simulink model "integration_LQR_model_4"  (R2023a)
settings: Solver=VariableStepAuto  StartTime=0.0  StopTime=30  FixedStep=SampleTime  RelTol=1e-3
PreLoadFcn:
  | %
  | 
  | %   Copyright 2020-2022 The MathWorks, Inc.
  | 
  | %Based on the quadcopter model used in jMAVSim
  | 
  | Ixx = 0.005; %Kgm^2
  | Iyy = 0.005;
  | Izz = 0.009;
  | 
  | 
  | inertia = diag([Ixx, Iyy, Izz]);
  | 
  | mass = 0.8; %Kg
  | g = 9.81; %m/s^2
  | 
  | armLength = 0.33/2; % length of Arm measured from center in m
  | 
  | rotorThrustMax = 4; %N
  | 
  | rotorTorqueMax = 0.05 ;%Nm
  | 
  | rotorTimeConst = 0.005 ;% time constant of rotor (motor + propeller)
  | 
  | %rotorOffset = [0 0 0]; % Rotors position offsets from Gravity center
  | 
  | dragCoeffMov = 0.01; %drag coefficient for linear motion of quadcopter
  | windVel = [0 0 0]';
  | 
  | % Initial states
  | init.posNED = [0, 0, 0]; % m
  | init.vb = [0 0 0]'; %m/s
  | init.euler = [0, 0, 0]'; %Roll Pitch Yaw Rads
  | init.angRates = [0, 0, 0]; %rad/s
  | 
  | 
  | %Computed from above values
  | rotorPositions = zeros(3,4);
  | axisD = armLength/sqrt(2);
  | rotorPositions(:,1) = [axisD, axisD, 0]';
  | rotorPositions(:,2) = [-axisD, -axisD, 0]';
  | rotorPositions(:,3) = [+axisD, -axisD, 0]';
  | rotorPositions(:,4) = [-axisD, axisD, 0]';
  | rotorDir = [-1, -1, 1, 1]; %rotation direction. +ve = clockwise
  | 
  | % Sample Time
  | SampleTime = 0.008;
  | 
  | %Gain to convert m to mm
  | m_to_mm = 1000;
  | 
  | %Gain to convert m/s^2 to mG
  | ms2_to_mg = (1/9.80665)*1000;
  | 
  | %Gain to convert m/s to cm/s
  | ms_to_cms = 100;
  | 
  | %Reference height for 'Flat Earth to LLA'
  | ref_height = -71.3232;
  | 
  | altToPrsGain = 12.0173;
  | altToPrsBias = 101270.95;
  | 
  | % Contact model
  | contact.translation.spring = 3100;
  | contact.translation.damper = 100;
  | contact.translation.friction = 0.5;
  | contact.translation.vd = 0.02;
  | contact.translation.maxFriction = 20;
  | contact.translation.maxNormal = 80;
  | 
  | contact.rotation.spring = 2;
  | contact.rotation.damper = 1;
  | contact.rotation.friction = 0.03;
  | control.rotation.maxMoment = 0.1;
  | control.rotation.friction = 0.025;
  | control.rotation.vd = 0.2;
  | 
  | 
  | %#######################################################
  | % Plant parameters
  | 
  | % Parameters for quadcopter_package_delivery
  | % Copyright 2021-2023 The MathWorks, Inc.
  | 
  | % Size of the ground
  | planex = 12.5;           % m
  | planey = 8.5;            % m
  | planedepth = 0.2;        % m, distance from plane to the reference frame
  | 
  | % Battery Capacity
  | battery_capacity = 7.6*3;
  | 
  | %% Material Property
  | % Assuming the arm of the drone is manufractured by 3D Printing, the ideal
  | % material is PLA, safe, light and cheap, the only concern is its thermal
  | % property
  | rho_pla   = 1.25;            % g/cm^3
  | 
  | % Measured drone mass
  | drone_mass = 1.2726;
  | %% package ground contact properties
  | pkgGrndStiff  = 1000;
  | pkgGrndDamp   = 300;
  | pkgGrndTransW = 1e-3;
  | 
  | 
  | %% Package parameters
  | pkgSize = [1 1 1]*0.14; % m
  | pkgDensity = 1/(pkgSize(1)*pkgSize(2)*pkgSize(3)); % kg/m^3
  | 
  | %% Propeller parameters
  | propeller.diameter = 0.254; % m
  | propeller.Kthrust  = 0.1072;
  | propeller.Kdrag    = 0.01;
  | 
  | air_rho            = 1.225;  % kg/m^3
  | air_temperature    = 273+25; % degK
  | wind_speed         = 0;      % Wind speed (m/s)
  | 
  | %% Leg parameters
  | drone_leg.Extr_Data = flipud([...
  |     0     0;
  |     0.5   0;
  |     1    -1;
  |     0.98 -1;
  |     0.5  -0.02;
  |    -0.5  -0.02;
  |    -0.98 -1;
  |    -1    -1;
  |    -0.5   0].*[1 1]*0.15);
  | 
  | drone_leg.width = 0.01;
  | 
  | %% Motor parameters
  | qc_motor.max_torque = 0.8;  % N*m
  | qc_motor.max_power  = 160;  % W
  | qc_motor.time_const = 0.02; % sec
  | qc_motor.efficiency = 25/30*100; % 0-100
  | qc_motor.efficiency_spd = 5000; % rpm
  | qc_motor.efficiency_trq = 0.05; % N*m
  | qc_motor.rotor_damping  = 1e-7; % N*m/(rad/s)
  | 
  | qc_max_power = qc_motor.max_power;
  | 
  | %% Controller parameters
  | filtM_position = 0.005;
  | kp_position    = 8;
  | ki_position    = 0.04;
  | kd_position    = 3.2;
  | filtD_position = 100;
  | pos2attitude   = 2.4;
  | 
  | filtM_attitude = 0.01;
  | kp_attitude    = 128.505;
  | ki_attitude    = 5.9203;
  | kd_attitude    = 78.2000*2;
  | filtD_attitude = 1000;
  | limit_attitude = 800;
  | 
  | filtM_yaw      = 0.01;
  | kp_yaw         = 25.7010*4*2;
  | ki_yaw         = 5.9203*0.01;
  | kd_yaw         = 78.2000*0.01;
  | filtD_yaw      = 100;
  | limit_yaw      = 20;
  | 
  | filtM_altitude = 0.05;
  | kp_altitude    = 0.27;
  | ki_altitude    = 0.07;
  | kd_altitude    = 0.35;
  | filtD_altitude = 10000;
  | limit_altitude = 10;
  | 
  | kp_motor       = 0.00375;
  | ki_motor       = 4.50000e-4;
  | kd_motor       = 0;
  | filtD_motor    = 10000;
  | filtSpd_motor    = 0.001;
  | limit_motor    = 0.25;
  | 
  | %% Drag coefficients
  | qd_drag.Cd_X = 0.35;
  | qd_drag.Cd_Y = 0.35;
  | qd_drag.Cd_Z = 0.6;
  | qd_drag.Roll = 0.2;
  | qd_drag.Pitch = 0.2;
  | qd_drag.Yaw = 0.2;
  | qd_area.YZ = 0.0875;
  | qd_area.XZ = 0.0900;
  | qd_area.XY = 0.2560;
  | qd_area.Roll = qd_area.XY*2;
  | qd_area.Pitch = qd_area.XY*2;
  | qd_area.Yaw = qd_area.XY;
  | 
  | 
  | waypoints = [-2,-2,0,2,5;-2,-2,0,0,0;0.14,6,6,6,0.14];
values from neighbouring files (symbols this model uses):
  delay_tilt = 0.004    [integration_parameters.m]    (also in simulation_parameters.m)
  kf = 65    [integration_parameters.m]    (also in simulation_parameters.m)
  Lh = 0.2    [CoG_shift.m]    (also in integration_parameters.m; simulation_parameters.m)
  Lv = 0.2    [integration_parameters.m]    (also in simulation_parameters.m)
  m = 1.12    [integration_parameters.m]    (also in optimal_controller_pitching.m; simulation_parameters.m)
  N = 150    [MPC_controller_full.m]
  reference = [1 1 1 0 30 40]'    [integration_parameters.m]    (also in simulation_parameters.m)
  roll_D = 1    [controller_parameters.m]    (also in integration_parameters.m)
  roll_I = 0    [controller_parameters.m]    (also in integration_parameters.m)
  roll_P = 8    [controller_parameters.m]    (also in integration_parameters.m)
  s_r = [1 1 1 1 1 1]    [integration_parameters.m]    (also in simulation_parameters.m)
  Tmax = 5.5    [integration_parameters.m]    (also in simulation_parameters.m)
  toll = 1e-12    [integration_parameters.m]    (also in simulation_parameters.m)
  vy_D = 0    [controller_parameters.m]    (also in integration_parameters.m)
  vy_I = 0    [controller_parameters.m]    (also in integration_parameters.m)
  vy_P = 12    [controller_parameters.m]    (also in integration_parameters.m)
  vz_D = 0    [controller_parameters.m]    (also in integration_parameters.m)
  vz_I = 0    [controller_parameters.m]    (also in integration_parameters.m = 1.5)
  vz_P = 8    [controller_parameters.m]    (also in integration_parameters.m = 9)
  y_D = 0.3    [controller_parameters.m]    (also in integration_parameters.m = 0)
  y_I = 0    [controller_parameters.m]    (also in integration_parameters.m)
  y_P = 1.5    [controller_parameters.m]    (also in integration_parameters.m = 0.8)
  yaw_D = 0    [controller_parameters.m]    (also in integration_parameters.m)
  yaw_I = 0    [controller_parameters.m]    (also in integration_parameters.m)
  yaw_P = 1.5    [controller_parameters.m]    (also in integration_parameters.m)
  z_D = 0    [controller_parameters.m]    (also in integration_parameters.m)
  z_I = 0    [controller_parameters.m]    (also in integration_parameters.m)
  z_P = 3    [controller_parameters.m]    (also in integration_parameters.m = 2.5)
undefined symbols (not defined in the file or in its folder): K, X, Y, Z
libraries: sm_lib x47, nesl_utility x23, slpidlib x6, simulink x5, simulink_extras x3, SignalEditorBlockLib x1
(part 1 of 3)
settings Model: Creator=joshu  LastModifiedBy=and20

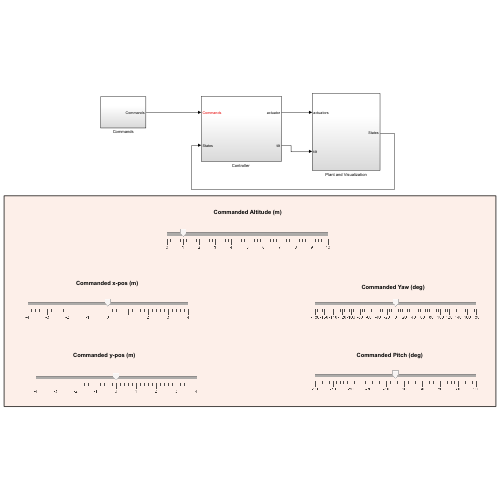
[thumbnail: Simulink's stored preview of the top-level diagram]
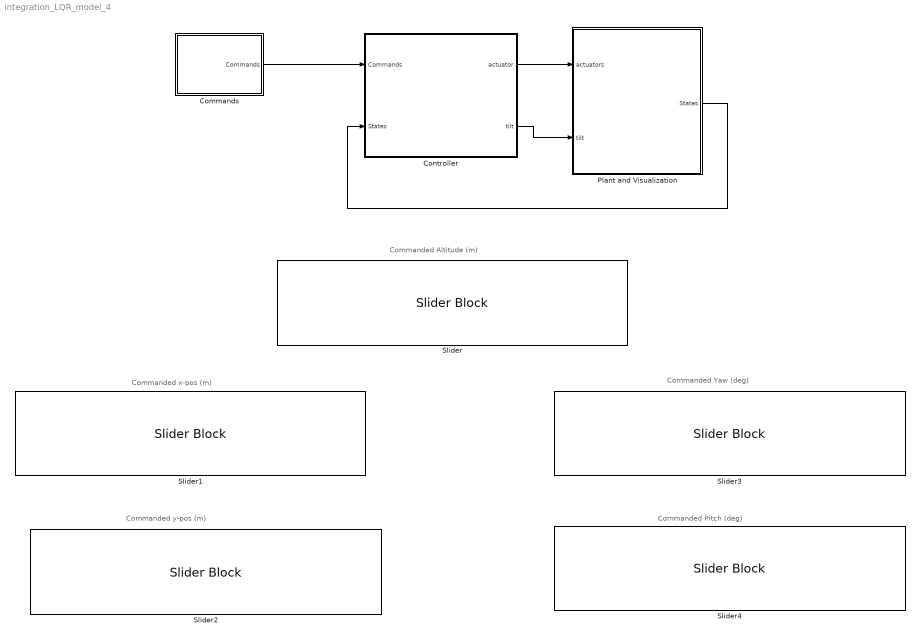
== system integration_LQR_model_4 ==
  note: Commanded Altitude (m)
  note: Commanded x-pos (m)
  note: Commanded y-pos (m)
  note: Commanded Yaw (deg)
  note: Commanded Pitch (deg)
  Commands : Subsystem
  "Controller " : Subsystem
  Plant and Visualization : Subsystem
  Slider : SliderBlock  LabelPosition=Hide  ScaleMax=10  TickInterval=1
  Slider1 : SliderBlock  LabelPosition=Hide  ScaleMin=-4  ScaleMax=4  TickInterval=1
  Slider2 : SliderBlock  LabelPosition=Hide  ScaleMin=-4  ScaleMax=4  TickInterval=1
  Slider3 : SliderBlock  LabelPosition=Hide  ScaleMin=-180  ScaleMax=180  TickInterval=20
  Slider4 : SliderBlock  LabelPosition=Hide  ScaleMin=-90  ScaleMax=90  TickInterval=20
  wires:
  Commands/1(Commands) -> "Controller "/1(Commands)
  Plant and Visualization/1(States) -> "Controller "/2(States)
  "Controller "/1(actuator) -> Plant and Visualization/1(actuators)
  "Controller "/2(tilt) -> Plant and Visualization/2(tilt)

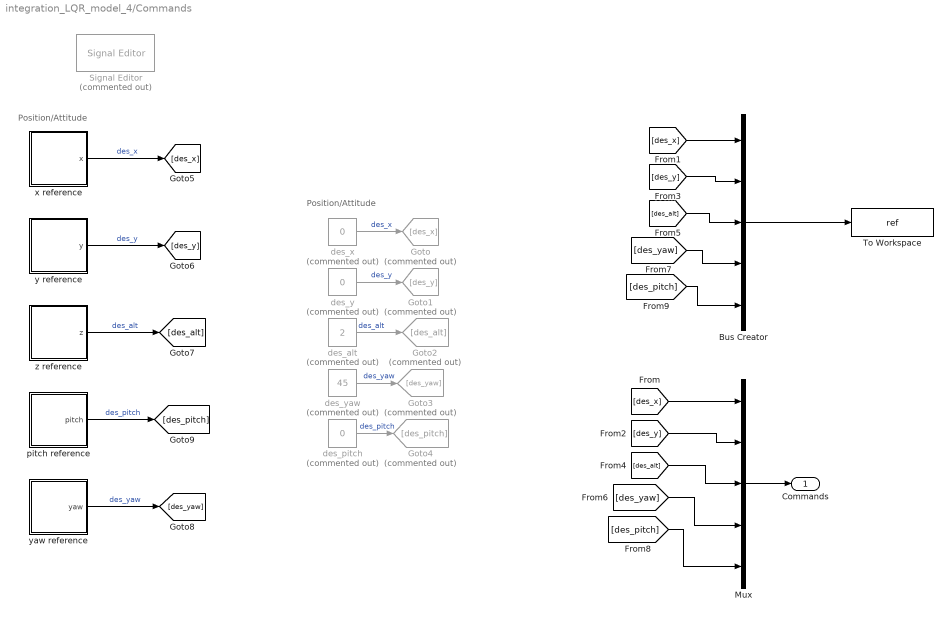
== system integration_LQR_model_4/Commands ==
  note: Position/Attitude
  note: Position/Attitude
  Bus Creator : BusCreator  Inputs=5
  Goto : Goto  Commented=on  GotoTag=des_x
  Goto1 : Goto  Commented=on  GotoTag=des_y
  Goto2 : Goto  Commented=on  GotoTag=des_alt
  Goto3 : Goto  Commented=on  GotoTag=des_yaw
  Goto4 : Goto  Commented=on  GotoTag=des_pitch
  Mux : Mux  Inputs=5
  Signal Editor : SignalEditorBlockLib/Signal Editor  Commented=on  FileName=reference_signal.mat  ActiveScenario=Scenario  ActiveSignal=x  IsBus=off  OutputBusObjectStr=Bus: BusObject  SampleTime=0  ZeroCross=off  OutputAfterFinalValue=Setting to zero  Unit=inherit  PreserveSignalName=on  ApplySigPropsToAllScenarios=on
  To Workspace : ToWorkspace  VariableName=ref  SaveFormat=Timeseries  SampleTime=-1
  des_alt : Constant  Commented=on  Value=2  SampleTime=SampleTime
  des_pitch : Constant  Commented=on  Value=0  SampleTime=SampleTime
  des_x : Constant  Commented=on  Value=0  SampleTime=SampleTime
  des_y : Constant  Commented=on  Value=0  SampleTime=SampleTime
  des_yaw : Constant  Commented=on  Value=45  SampleTime=SampleTime
  pitch reference : Subsystem
  x reference : Subsystem
  y reference : Subsystem
  yaw reference : Subsystem
  z reference : Subsystem
  Commands : Outport
  wires:
  Mux/1 -> Commands/1
  Bus Creator/1 -> To Workspace/1
  [des_x] -> Mux/1
  [des_x] -> Bus Creator/1
  [des_y] -> Mux/2
  [des_y] -> Bus Creator/2
  [des_alt] -> Mux/3
  [des_alt] -> Bus Creator/3
  [des_yaw] -> Mux/4
  [des_yaw] -> Bus Creator/4
  [des_pitch] -> Mux/5
  [des_pitch] -> Bus Creator/5
  des_x/1 -> Goto/1  "des_x"
  des_alt/1 -> Goto2/1  "des_alt"
  des_y/1 -> Goto1/1  "des_y"
  des_pitch/1 -> Goto4/1  "des_pitch"
  des_yaw/1 -> Goto3/1  "des_yaw"
  z reference/1(z) -> [des_alt]  "des_alt"
  yaw reference/1(yaw) -> [des_yaw]  "des_yaw"
  y reference/1(y) -> [des_y]  "des_y"
  x reference/1(x) -> [des_x]  "des_x"
  pitch reference/1(pitch) -> [des_pitch]  "des_pitch"

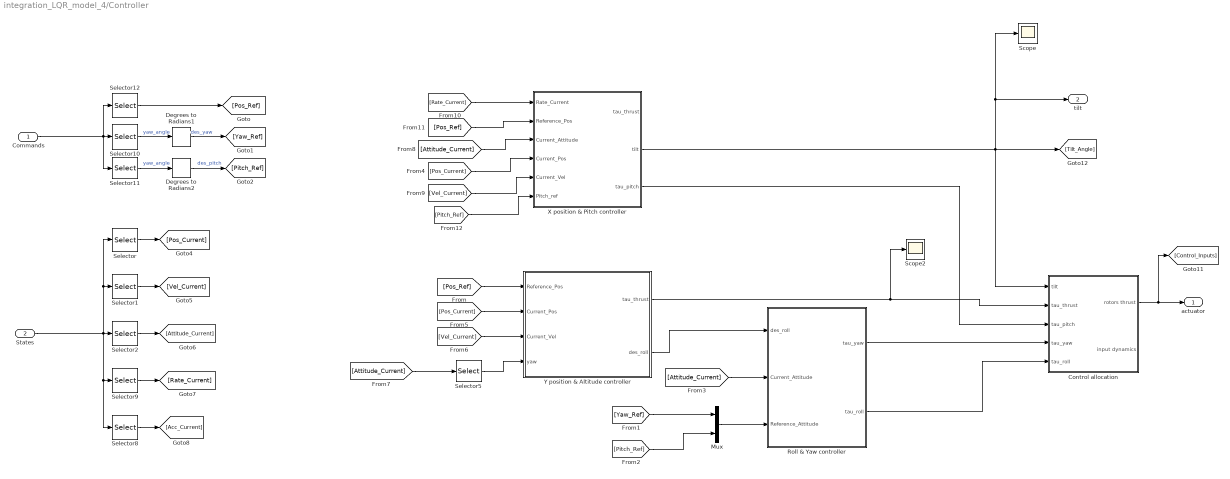
== system integration_LQR_model_4/Controller  ==
  Commands : Inport
  States : Inport  Port=2
  Control allocation : Subsystem
  Degrees to Radians1 : simulink_extras/Transformations/Degrees to Radians
  Degrees to Radians2 : simulink_extras/Transformations/Degrees to Radians
  Mux : Mux  Inputs=2
  Roll & Yaw controller : Subsystem
  Scope : Scope
  Scope2 : Scope
  Selector : Selector  InputPortWidth=15  IndexOptions=Index vector (dialog)  Indices=[1:3]  OutputSizes=1
  Selector1 : Selector  InputPortWidth=15  IndexOptions=Index vector (dialog)  Indices=[7:9]  OutputSizes=1
  Selector10 : Selector  InputPortWidth=5  IndexOptions=Index vector (dialog)  Indices=4  OutputSizes=1
  Selector11 : Selector  InputPortWidth=5  IndexOptions=Index vector (dialog)  Indices=5  OutputSizes=1
  Selector12 : Selector  InputPortWidth=5  IndexOptions=Index vector (dialog)  Indices=[1 2 3]  OutputSizes=1
  Selector2 : Selector  InputPortWidth=15  IndexOptions=Index vector (dialog)  Indices=[4:6]  OutputSizes=1
  Selector5 : Selector  InputPortWidth=3  IndexOptions=Index vector (dialog)  Indices=3  OutputSizes=1
  Selector8 : Selector  InputPortWidth=15  IndexOptions=Index vector (dialog)  Indices=[13:15]  OutputSizes=1
  Selector9 : Selector  InputPortWidth=15  IndexOptions=Index vector (dialog)  Indices=[10:12]  OutputSizes=1
  X position & Pitch controller : Subsystem
  Y position & Altitude controller : Subsystem
  actuator : Outport
  tilt : Outport  Port=2
  wires:
  States/1 -> Selector1/1, Selector/1, Selector8/1, Selector9/1, Selector2/1
  Selector2/1 -> [Attitude_Current]
  Selector10/1 -> Degrees to Radians1/1  "yaw_angle"
  Selector11/1 -> Degrees to Radians2/1  "yaw_angle"
  Commands/1 -> Selector11/1, Selector12/1, Selector10/1
  Selector12/1 -> [Pos_Ref]
  Degrees to Radians1/1 -> [Yaw_Ref]  "des_yaw"
  Degrees to Radians2/1 -> [Pitch_Ref]  "des_pitch"
  Selector/1 -> [Pos_Current]
  Selector1/1 -> [Vel_Current]
  Selector9/1 -> [Rate_Current]
  Selector8/1 -> [Acc_Current]
  Y position & Altitude controller/2(des_roll) -> Roll & Yaw controller/1(des_roll)
  X position & Pitch controller/2(tilt) -> Scope/1, tilt/1, Control allocation/1(tilt), [Tilt_Angle]
  [Yaw_Ref] -> Mux/1
  [Pitch_Ref] -> Mux/2
  [Attitude_Current] -> Selector5/1
  [Pos_Ref] -> Y position & Altitude controller/1(Reference_Pos)
  [Pos_Current] -> Y position & Altitude controller/2(Current_Pos)
  [Vel_Current] -> Y position & Altitude controller/3(Current_Vel)
  Selector5/1 -> Y position & Altitude controller/4(yaw)
  [Attitude_Current] -> X position & Pitch controller/3(Current_Attitude)
  [Attitude_Current] -> Roll & Yaw controller/2(Current_Attitude)
  Mux/1 -> Roll & Yaw controller/3(Reference_Attitude)
  Control allocation/1(rotors thrust) -> [Control_Inputs], actuator/1
  Y position & Altitude controller/1(tau_thrust) -> Scope2/1, Control allocation/2(tau_thrust)
  X position & Pitch controller/3(tau_pitch) -> Control allocation/3(tau_pitch)
  Roll & Yaw controller/1(tau_yaw) -> Control allocation/4(tau_yaw)
  Roll & Yaw controller/2(tau_roll) -> Control allocation/5(tau_roll)
  [Pos_Current] -> X position & Pitch controller/4(Current_Pos)
  [Vel_Current] -> X position & Pitch controller/5(Current_Vel)
  [Rate_Current] -> X position & Pitch controller/1(Rate_Current)
  [Pos_Ref] -> X position & Pitch controller/2(Reference_Pos)
  [Pitch_Ref] -> X position & Pitch controller/6(Pitch_ref)

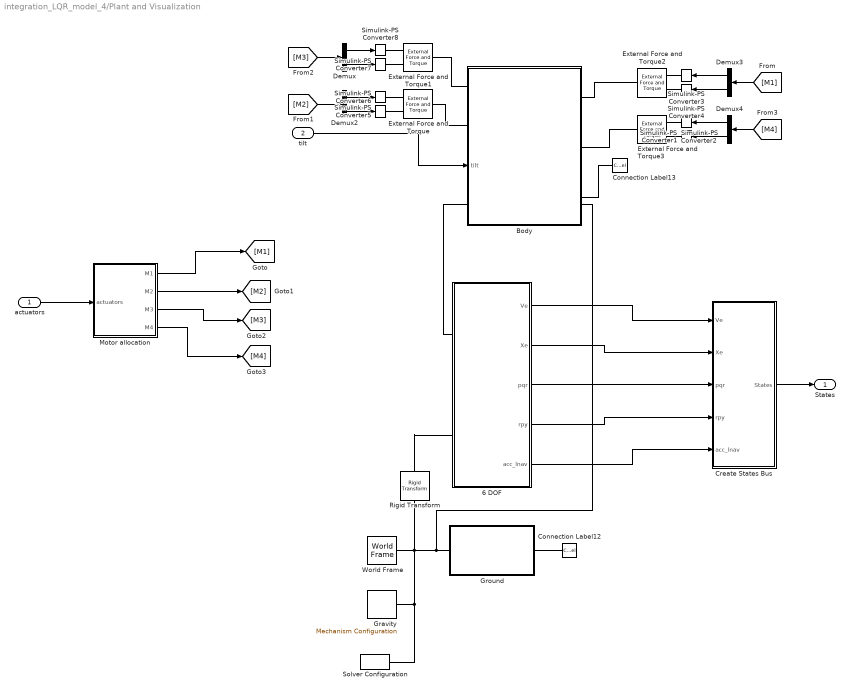
== system integration_LQR_model_4/Plant and Visualization ==
  actuators : Inport
  tilt : Inport  Port=2
  6 DOF : Subsystem
  Body : Subsystem
      settings: PortSchema="{\"entries\":[{\"content\":{\"sides\":[{\"content\":{\"connectorIds\":[\"LConn1\",\"LConn2\",\"In1\",\"LConn3\"]},\"type\":\"ConnectorPlacement.EquallySpacedRectSide\",\"uuid\":\"ae3cb6d2-0ab8-4029-8c07-9e22db9f1c51\"},{\"content\":{\"connectorIds\":[\"RConn1\",\"RConn2\",\"RConn3\"],\"side\":\"RIGHT\"},\"type\":\"ConnectorPlacement.EquallySpacedRectSide\",\"uuid\":\"2ad5b30e-93e6-4417-a12e-628dc0d83472\"},{\"content\":{\"side\":\"TOP\"},\"type\":\"ConnectorPlacement.EquallySpacedRectSide\",\"uuid\":\"9a1538ce-9fff-476b-ad69-664f8ff19368\"}]},\"type\":\"ConnectorPlacement.EquallySpacedConnector\",\"uuid\":\"2220cfc5-a376-4ffb-9762-6061b092de10\"}],\"packageUris\":[\"http://schema.mathworks.com/mf0/Connector/R2020b\"],\"version\":\"1.0\"}"
  Connection Label12 : ConnectionLabel  Label=G
  Connection Label13 : ConnectionLabel  Label=G
  Create States Bus : Subsystem
  Demux{,2..4} (4 alike) : Demux  Outputs=2
  External Force and Torque{,1..3} (4 alike) : sm_lib/Forces and Torques/External Force and Torque  ForceResolutionFrame=AttachedFrame  EnableForceX=off  EnableForceY=on  EnableForceZ=off  EnableForce=off  TorqueResolutionFrame=AttachedFrame  EnableTorqueX=off  EnableTorqueY=on  EnableTorqueZ=off  EnableTorque=off
  Gravity : sm_lib/Utilities/Mechanism Configuration  UniformGravity=Constant  GravityVector=[0 0 -9.80665]  GravityVectorUnits=m/s^2  LinearizationDelta=0.001  JointModeTransitionNonlinearIterations=2
  Ground : Subsystem
  Motor allocation : Subsystem
  Rigid Transform : sm_lib/Frames and Transforms/Rigid Transform  TranslationMethod=StandardAxis  TranslationStandardOffset=0.15  TranslationStandardOffsetUnits=m  TranslationStandardAxis=+Z  TranslationCartesianOffset=[0 0 0]  TranslationCartesianOffsetUnits=m  TranslationROffset=0  TranslationROffsetUnits=m  TranslationZOffset=0  TranslationZOffsetUnits=m  TranslationThetaOffset=0  TranslationThetaOffsetUnits=deg  RotationMethod=None  RotationAngleUnits=deg  RotationStandardAxis=+X  RotationAngle=180  RotationArbitraryAxis=[0 0 1]  FollAlignAxisA=+X  BaseAlignAxisA=+Y  FollAlignAxisB=+Y  BaseAlignAxisB=+Z  RotationSequenceAxes=FollowerAxes  RotationSequence=XYX  RotationSequenceAngles=[0 0 0]  RotationSequenceAnglesUnits=deg  RotationMatrix=[1 0 0; 0 1 0; 0 0 1]  Quaternion=[1 0 0 0]
  Simulink-PS Converter{1..8} (8 alike) : nesl_utility/Simulink-PS Converter  PhysicalDomain=network_engine_domain  SubClassName=ps_input  LeftPortType=input  RightPortType=output  PseudoPeriodic=off  Frequencies=[]  NoiseDistribution=none  NoiseParameters=[]  Unit=1  AffineConversion=off  FilteringAndDerivatives=filter  SimscapeFilterOrder=2  InputFilterTimeConstant=0.001  UdotUserProvided=0
  Solver Configuration : nesl_utility/Solver Configuration  PhysicalDomain=network_engine_domain  SubClassName=solver  LeftPortType=input  RightPortType=generic  Tones=[]  Harmonics=[]  SimulateNoise=off  Profile=off  UseLocalSampling=off  EnableSwitchedLinearOptims=on  FrequencyDomain=off  UseCCode=off  RelTol=0.001  AbsTol=1e-06  MinStep=1e-09  ToWorkspace=off  RevertToSquareIcSolve=off  NumHomotopyIterations=100  PhasorMode=off  PhasorModeNumHarmonics=1  ConsistencySolver=NEWTON_FTOL  IndexReductionMethod=DerivativeReplacement  DoDC=off  ResidualTolerance=1e-9  ConsistencyTolSource=GLOBAL  ConsistencyAbsTol=0.001  ConsistencyRelTol=0.001  ConsistencyTolFactor=0.001  UseLocalSolver=off  LocalSolverChoice=NE_BACKWARD_EULER_ADVANCER  ResolveIndetEquations=on  FunctionEvalNumThread=1  LocalSolverSampleTime=0.01  DoFixedCost=off  MaxNonlinIter=2  MaxModeIter=2  ComputeImpulses=off  ImpulseIterations=2  LinearAlgebra=auto  LinearAlgebraNumThread=0  EquationFormulation=NE_TIME_EF  DelaysMemoryBudget=1024  AutomaticFiltering=on  FilteringTimeConstant=0.001  PartitionStorageMethod=AS_NEEDED  PartitionMemoryBudget=1024  PartitionMethod=FAST
  World Frame : sm_lib/Frames and Transforms/World Frame
  States : Outport
  wires:
  Create States Bus/1(States) -> States/1
  [M1] -> Demux3/1
  Demux4/1 -> Simulink-PS Converter2/1
  [M3] -> Demux/1
  Demux3/2 -> Simulink-PS Converter4/1
  Demux/2 -> Simulink-PS Converter7/1
  6 DOF/5(acc_lnav) -> Create States Bus/5(acc_lnav)
  6 DOF/3(pqr) -> Create States Bus/3(pqr)
  6 DOF/4(rpy) -> Create States Bus/4(rpy)
  6 DOF/2(Xe) -> Create States Bus/2(Xe)
  6 DOF/1(Ve) -> Create States Bus/1(Ve)
  [M4] -> Demux4/1
  Demux2/2 -> Simulink-PS Converter5/1
  [M2] -> Demux2/1
  Demux3/1 -> Simulink-PS Converter3/1
  Demux2/1 -> Simulink-PS Converter6/1
  Demux/1 -> Simulink-PS Converter8/1
  Demux4/2 -> Simulink-PS Converter1/1
  tilt/1 -> Body/1(tilt)
  actuators/1 -> Motor allocation/1(actuators)
  Motor allocation/1(M1) -> [M1]
  Motor allocation/2(M2) -> [M2]
  Motor allocation/3(M3) -> [M3]
  Motor allocation/4(M4) -> [M4]
  connections:
  External Force and Torque2/LConn1 -- Simulink-PS Converter3/RConn1
  External Force and Torque3/RConn1 -- Body/RConn2
  Connection Label12/LConn1 -- Ground/LConn1
  External Force and Torque2/RConn1 -- Body/RConn1
  Connection Label13/LConn1 -- Body/RConn3
  Simulink-PS Converter8/RConn1 -- External Force and Torque1/LConn1
  External Force and Torque/RConn1 -- Body/LConn2
  External Force and Torque3/LConn1 -- Simulink-PS Converter2/RConn1
  Simulink-PS Converter7/RConn1 -- External Force and Torque1/LConn2
  External Force and Torque1/RConn1 -- Body/LConn1
  Simulink-PS Converter6/RConn1 -- External Force and Torque/LConn1
  Simulink-PS Converter5/RConn1 -- External Force and Torque/LConn2
  External Force and Torque2/LConn2 -- Simulink-PS Converter4/RConn1
  External Force and Torque3/LConn2 -- Simulink-PS Converter1/RConn1
  Body/LConn3 -- 6 DOF/LConn1
  Rigid Transform/RConn1 -- 6 DOF/LConn2
  World Frame/RConn1 -- Rigid Transform/LConn1 -- Solver Configuration/RConn1 -- Gravity/RConn1 -- Ground/RConn1

== system integration_LQR_model_4/Commands/pitch reference ==
  note: 0 for step
      | 1 for ramp
  Constant : Constant  Value=s_r(5)
  Ramp1 : simulink/Sources/Ramp  slope=180/pi/4  start=25  InitialOutput=0
  Saturation1 : Saturate  UpperLimit=abs(reference(5))  LowerLimit=-abs(reference(5))
  Step : Step  Time=10  After=reference(5)  SampleTime=0
  Switch : Switch  Criteria=u2 > Threshold  SaturateOnIntegerOverflow=off  InputSameDT=off
  pitch : Outport
  wires:
  Ramp1/1 -> Saturation1/1
  Saturation1/1 -> Switch/1
  Switch/1 -> pitch/1
  Constant/1 -> Switch/2
  Step/1 -> Switch/3

== system integration_LQR_model_4/Commands/x reference ==
  note: 0 for step
      | 1 for ramp
  Constant : Constant  Value=s_r(1)
  Ramp1 : simulink/Sources/Ramp  slope=1  start=15  InitialOutput=0
  Saturation1 : Saturate  UpperLimit=abs(reference(1))  LowerLimit=-abs(reference(1))
  Step : Step  Time=10  After=reference(1)  SampleTime=0
  Switch : Switch  Criteria=u2 > Threshold  SaturateOnIntegerOverflow=off  InputSameDT=off
  x : Outport
  wires:
  Ramp1/1 -> Saturation1/1
  Saturation1/1 -> Switch/1
  Switch/1 -> x/1
  Constant/1 -> Switch/2
  Step/1 -> Switch/3

== system integration_LQR_model_4/Commands/y reference ==
  note: 0 for step
      | 1 for ramp
  Constant1 : Constant  Value=s_r(2)
  Ramp2 : simulink/Sources/Ramp  slope=1  start=20  InitialOutput=0
  Saturation2 : Saturate  UpperLimit=abs(reference(2))  LowerLimit=-abs(reference(2))
  Step : Step  Time=10  After=reference(2)  SampleTime=0
  Switch1 : Switch  Criteria=u2 > Threshold  SaturateOnIntegerOverflow=off  InputSameDT=off
  y : Outport
  wires:
  Step/1 -> Switch1/3
  Ramp2/1 -> Saturation2/1
  Constant1/1 -> Switch1/2
  Saturation2/1 -> Switch1/1
  Switch1/1 -> y/1

== system integration_LQR_model_4/Commands/yaw reference ==
  note: 0 for step
      | 1 for ramp
  Constant1 : Constant  Value=s_r(6)
  Ramp2 : simulink/Sources/Ramp  slope=180/pi/4  start=10  InitialOutput=0
  Saturation2 : Saturate  UpperLimit=abs(reference(6))  LowerLimit=-abs(reference(6))
  Step : Step  Time=10  After=reference(6)  SampleTime=0
  Switch1 : Switch  Criteria=u2 > Threshold  SaturateOnIntegerOverflow=off  InputSameDT=off
  yaw : Outport
  wires:
  Step/1 -> Switch1/3
  Ramp2/1 -> Saturation2/1
  Constant1/1 -> Switch1/2
  Saturation2/1 -> Switch1/1
  Switch1/1 -> yaw/1

== system integration_LQR_model_4/Commands/z reference ==
  note: 0 for step
      | 1 for ramp
  Constant : Constant  Value=s_r(3)
  Ramp1 : simulink/Sources/Ramp  slope=1  start=5  InitialOutput=0
  Saturation1 : Saturate  UpperLimit=abs(reference(3))  LowerLimit=-abs(reference(3))
  Step : Step  Time=10  After=reference(3)  SampleTime=0
  Switch : Switch  Criteria=u2 > Threshold  SaturateOnIntegerOverflow=off  InputSameDT=off
  z : Outport
  wires:
  Ramp1/1 -> Saturation1/1
  Step/1 -> Switch/3
  Saturation1/1 -> Switch/1
  Switch/1 -> z/1
  Constant/1 -> Switch/2

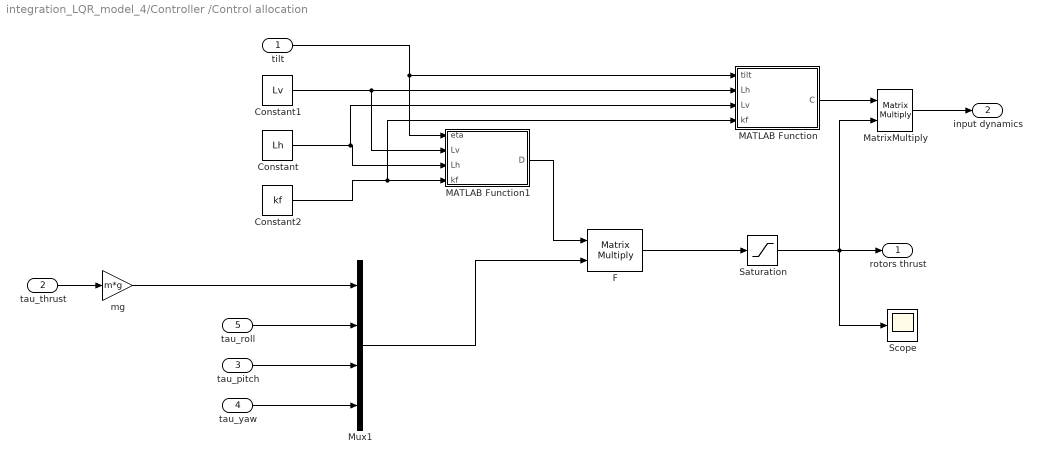
== system integration_LQR_model_4/Controller /Control allocation ==
  tilt : Inport
  tau_thrust : Inport  Port=2
  tau_pitch : Inport  Port=3
  tau_yaw : Inport  Port=4
  tau_roll : Inport  Port=5
  Constant : Constant  Value=Lh
  Constant1 : Constant  Value=Lv
  Constant2 : Constant  Value=kf
  F : Product  Multiplication=Matrix(*)
  MATLAB Function : MATLAB Function  TreatAsAtomicUnit=on
  MATLAB Function1 : MATLAB Function  TreatAsAtomicUnit=on
  MatrixMultiply : Product  Multiplication=Matrix(*)
  Mux1 : Mux
  Saturation : Saturate  UpperLimit=Tmax  LowerLimit=0
  Scope : Scope
  mg : Gain  Gain=m*g
  rotors thrust : Outport
  input dynamics : Outport  Port=2
  wires:
  tau_thrust/1 -> mg/1
  tau_pitch/1 -> Mux1/3
  mg/1 -> Mux1/1
  Constant1/1 -> MATLAB Function/2(Lh), MATLAB Function1/2(Lv)
  MATLAB Function1/1(D) -> F/1
  Constant/1 -> MATLAB Function/3(Lv), MATLAB Function1/3(Lh)
  Constant2/1 -> MATLAB Function/4(kf), MATLAB Function1/4(kf)
  Mux1/1 -> F/2
  F/1 -> Saturation/1
  tilt/1 -> MATLAB Function1/1(eta), MATLAB Function/1(tilt)
  Saturation/1 -> Scope/1, MatrixMultiply/2, rotors thrust/1
  MATLAB Function/1(C) -> MatrixMultiply/1
  MatrixMultiply/1 -> input dynamics/1
  tau_yaw/1 -> Mux1/4
  tau_roll/1 -> Mux1/2

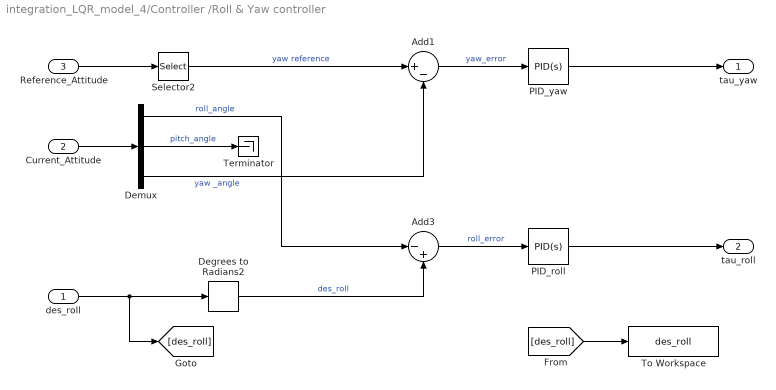
== system integration_LQR_model_4/Controller /Roll & Yaw controller ==
  des_roll : Inport
  Current_Attitude : Inport  Port=2
  Reference_Attitude : Inport  Port=3
  Add1 : Sum  Inputs=|+-
  Add3 : Sum  Inputs=|-+
  Degrees to Radians2 : simulink_extras/Transformations/Degrees to Radians
  Demux : Demux  Outputs=3
  PID_roll : slpidlib/PID Controller  Controller=PID  Form=Parallel  TimeDomain=Continuous-time  UseExternalTs=off  SampleTime=-1  IntegratorMethod=Backward Euler  FilterMethod=Forward Euler  ControllerParametersSource=internal  P=roll_P  I=roll_I  UseKiTs=off  D=roll_D  N=100  UseFilter=on  TunerSelectOption=Transfer Function Based (PID Tuner App)  InitialConditionSource=internal  InitialConditionForIntegrator=0  InitialConditionForFilter=0  DifferentiatorICPrevScaledInput=0  ExternalReset=none  TrackingMode=off  Kt=1  LimitOutput=off  SatLimitsSource=internal  UpperSaturationLimit=0.05  LowerSaturationLimit=-0.05  LinearizeAsGain=off  AntiWindupMode=none  Kb=1  LimitIntegrator=off  UpperIntegratorSaturationLimit=inf  LowerIntegratorSaturationLimit=-inf  POutMin=[]  POutMax=[]  IOutMin=[]  IOutMax=[]  DOutMin=[]  DOutMax=[]  NOutMin=[]  NOutMax=[]  SumOutMin=[]  SumOutMax=[]  SaturationOutMin=[]  SaturationOutMax=[]  PParamMin=[]  PParamMax=[]  IParamMin=[]  IParamMax=[]  DParamMin=[]  DParamMax=[]  NParamMin=[]  NParamMax=[]  KbParamMin=[]  KbParamMax=[]  KtParamMin=[]  KtParamMax=[]  KbOutMin=[]  KbOutMax=[]  KtOutMin=[]  KtOutMax=[]  IntegratorOutMin=[]  IntegratorOutMax=[]  FilterOutMin=[]  FilterOutMax=[]  SumI1OutMin=[]  SumI1OutMax=[]  SumI2OutMin=[]  SumI2OutMax=[]  SumI3OutMin=[]  SumI3OutMax=[]  SumI4OutMin=[]  SumI4OutMax=[]  SumDOutMin=[]  SumDOutMax=[]  DifferentiatorOutMin=[]  DifferentiatorOutMax=[]  FilterDiffOutCoefMin=[]  FilterDiffOutCoefMax=[]  ReciprocalOutMin=[]  ReciprocalOutMax=[]  SumDenOutMin=[]  SumDenOutMax=[]  SumNumOutMin=[]  SumNumOutMax=[]  DivideOutMin=[]  DivideOutMax=[]  UdiffTsProdOutMin=[]  UdiffTsProdOutMax=[]  NTsProdOutMin=[]  NTsProdOutMax=[]  UintegralTsProdOutMin=[]  UintegralTsProdOutMax=[]  UngainTsProdOutMin=[]  UngainTsProdOutMax=[]  ClampingZeroOutDataTypeStr=Inherit: Inherit via back propagation  ClampingZeroOutMin=[]  ClampingZeroOutMax=[]  FilterDenConstantOutDataTypeStr=Inherit: Inherit via back propagation  FilterDenConstantOutMin=[]  FilterDenConstantOutMax=[]  PCopyOutDataTypeStr=Inherit: Inherit via back propagation  PCopyOutMin=[]  PCopyOutMax=[]  NCopyOutDataTypeStr=Inherit: Inherit via back propagation  NCopyOutMin=[]  NCopyOutMax=[]  IntegratorContinuousStateAttributes=''  IntegratorStateMustResolveToSignalObject=off  IntegratorRTWStateStorageClass=Auto  FilterContinuousStateAttributes=''  FilterStateMustResolveToSignalObject=off  FilterRTWStateStorageClass=Auto  ParallelPVariant=InternalParameters  IdealPVariant=Disabled  IVariant=InternalParameters  DVariant=InternalParameters  IntegratorVariant=Continuous  SatVariant=Disabled  AWVariant=Passthrough  PCopyVariant=Disabled  TRVariant=Disabled  FdbkBlocksVariant=Forward  IdealPFdbkVariant=Disabled  SatFdbkVariant=Disabled  DerivativeFilterVariant=ContFilter  NVariant=InternalParameters  NCopyVariant=Disabled  FilterICVariant=InternalICsFilter  IntegratorICVariant=InternalICs  ExternalResetVariant=Disabled  TRSumVariant=Passthrough  SumFdbkVariant=Disabled  SumVariant=Sum_PID  TsampFilterVariant=InternalTs  TsampNgainVariant=Passthrough  TsampIntegralVariant=Disabled_SignalSpec  ExternalSaturationOutDataTypeStr=Inherit: Same as second input
  PID_yaw : slpidlib/PID Controller  Controller=PID  Form=Parallel  TimeDomain=Continuous-time  UseExternalTs=off  SampleTime=-1  IntegratorMethod=Backward Euler  FilterMethod=Forward Euler  ControllerParametersSource=internal  P=yaw_P  I=yaw_I  UseKiTs=off  D=yaw_D  N=100  UseFilter=on  TunerSelectOption=Transfer Function Based (PID Tuner App)  InitialConditionSource=internal  InitialConditionForIntegrator=0  InitialConditionForFilter=0  DifferentiatorICPrevScaledInput=0  ExternalReset=none  TrackingMode=off  Kt=1  LimitOutput=off  SatLimitsSource=internal  UpperSaturationLimit=0.01  LowerSaturationLimit=-0.01  LinearizeAsGain=off  AntiWindupMode=clamping  Kb=1  LimitIntegrator=off  UpperIntegratorSaturationLimit=inf  LowerIntegratorSaturationLimit=-inf  POutMin=[]  POutMax=[]  IOutMin=[]  IOutMax=[]  DOutMin=[]  DOutMax=[]  NOutMin=[]  NOutMax=[]  SumOutMin=[]  SumOutMax=[]  SaturationOutMin=[]  SaturationOutMax=[]  PParamMin=[]  PParamMax=[]  IParamMin=[]  IParamMax=[]  DParamMin=[]  DParamMax=[]  NParamMin=[]  NParamMax=[]  KbParamMin=[]  KbParamMax=[]  KtParamMin=[]  KtParamMax=[]  KbOutMin=[]  KbOutMax=[]  KtOutMin=[]  KtOutMax=[]  IntegratorOutMin=[]  IntegratorOutMax=[]  FilterOutMin=[]  FilterOutMax=[]  SumI1OutMin=[]  SumI1OutMax=[]  SumI2OutMin=[]  SumI2OutMax=[]  SumI3OutMin=[]  SumI3OutMax=[]  SumI4OutMin=[]  SumI4OutMax=[]  SumDOutMin=[]  SumDOutMax=[]  DifferentiatorOutMin=[]  DifferentiatorOutMax=[]  FilterDiffOutCoefMin=[]  FilterDiffOutCoefMax=[]  ReciprocalOutMin=[]  ReciprocalOutMax=[]  SumDenOutMin=[]  SumDenOutMax=[]  SumNumOutMin=[]  SumNumOutMax=[]  DivideOutMin=[]  DivideOutMax=[]  UdiffTsProdOutMin=[]  UdiffTsProdOutMax=[]  NTsProdOutMin=[]  NTsProdOutMax=[]  UintegralTsProdOutMin=[]  UintegralTsProdOutMax=[]  UngainTsProdOutMin=[]  UngainTsProdOutMax=[]  ClampingZeroOutDataTypeStr=Inherit: Inherit via back propagation  ClampingZeroOutMin=[]  ClampingZeroOutMax=[]  FilterDenConstantOutDataTypeStr=Inherit: Inherit via back propagation  FilterDenConstantOutMin=[]  FilterDenConstantOutMax=[]  PCopyOutDataTypeStr=Inherit: Inherit via back propagation  PCopyOutMin=[]  PCopyOutMax=[]  NCopyOutDataTypeStr=Inherit: Inherit via back propagation  NCopyOutMin=[]  NCopyOutMax=[]  IntegratorContinuousStateAttributes=''  IntegratorStateMustResolveToSignalObject=off  IntegratorRTWStateStorageClass=Auto  FilterContinuousStateAttributes=''  FilterStateMustResolveToSignalObject=off  FilterRTWStateStorageClass=Auto  ParallelPVariant=InternalParameters  IdealPVariant=Disabled  IVariant=InternalParameters  DVariant=InternalParameters  IntegratorVariant=Continuous  SatVariant=Disabled  AWVariant=Passthrough  PCopyVariant=Disabled  TRVariant=Disabled  FdbkBlocksVariant=Forward  IdealPFdbkVariant=Disabled  SatFdbkVariant=Disabled  DerivativeFilterVariant=ContFilter  NVariant=InternalParameters  NCopyVariant=Disabled  FilterICVariant=InternalICsFilter  IntegratorICVariant=InternalICs  ExternalResetVariant=Disabled  TRSumVariant=Passthrough  SumFdbkVariant=Disabled  SumVariant=Sum_PID  TsampFilterVariant=InternalTs  TsampNgainVariant=Passthrough  TsampIntegralVariant=Disabled_SignalSpec  ExternalSaturationOutDataTypeStr=Inherit: Same as second input
  Selector2 : Selector  InputPortWidth=2  IndexOptions=Index vector (dialog)  Indices=[1]  OutputSizes=1
  Terminator : Terminator
  To Workspace : ToWorkspace  VariableName=des_roll  SaveFormat=Timeseries  SampleTime=-1
  tau_yaw : Outport
  tau_roll : Outport  Port=2
  wires:
  Add3/1 -> PID_roll/1  "roll_error"
  Add1/1 -> PID_yaw/1  "yaw_error"
  des_roll/1 -> [des_roll], Degrees to Radians2/1
  Degrees to Radians2/1 -> Add3/2  "des_roll"
  Selector2/1 -> Add1/1  "yaw reference"
  Reference_Attitude/1 -> Selector2/1
  Current_Attitude/1 -> Demux/1
  PID_yaw/1 -> tau_yaw/1
  PID_roll/1 -> tau_roll/1
  Demux/2 -> Terminator/1  "pitch_angle"
  Demux/3 -> Add1/2  "yaw _angle"
  Demux/1 -> Add3/1  "roll_angle"
  [des_roll] -> To Workspace/1

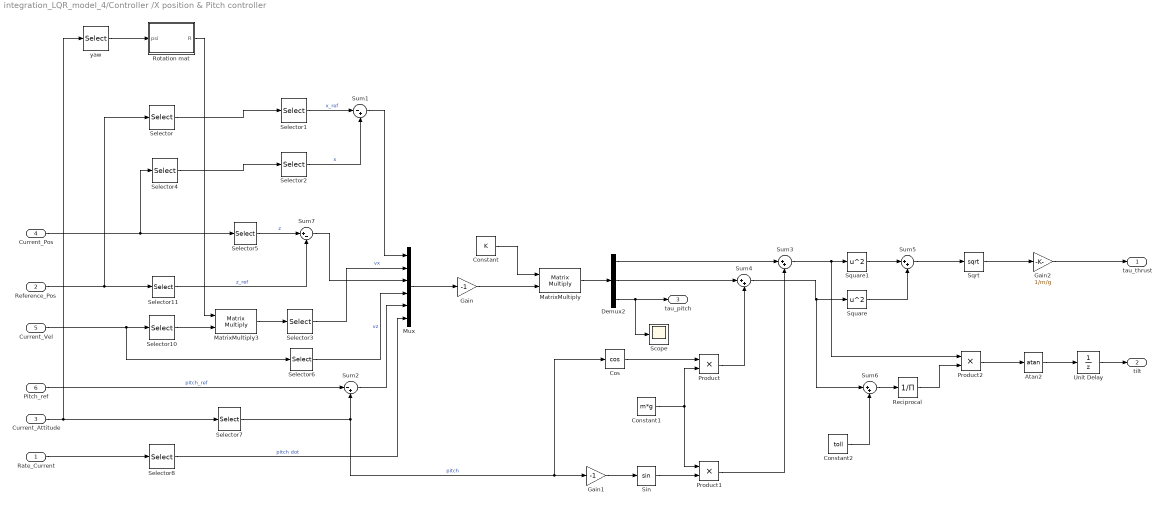
== system integration_LQR_model_4/Controller /X position & Pitch controller ==
  Rate_Current : Inport
  Reference_Pos : Inport  Port=2
  Current_Attitude : Inport  Port=3
  Current_Pos : Inport  Port=4
  Current_Vel : Inport  Port=5
  Pitch_ref : Inport  Port=6
  Atan2 : Trigonometry  Operator=atan
  Constant : Constant  Value=K  VectorParams1D=off
  Constant1 : Constant  Value=m*g
  Constant2 : Constant  Value=toll
  Cos : Trigonometry  Operator=cos
  Demux2 : Demux  Outputs=3
  Gain : Gain  Gain=-1
  Gain1 : Gain  Gain=-1
  Gain2 : Gain  Gain=1/m/g
  MatrixMultiply : Product  Multiplication=Matrix(*)
  MatrixMultiply3 : Product  Multiplication=Matrix(*)
  Mux : Mux  Inputs=6
  Product : Product
  Product1 : Product
  Product2 : Product
  Reciprocal : Product  Inputs=/
  "Rotation mat " : MATLAB Function  TreatAsAtomicUnit=on
  Scope : Scope
  Selector : Selector  InputPortWidth=3  IndexOptions=Index vector (dialog)  Indices=[1 2]  OutputSizes=1
  Selector1 : Selector  InputPortWidth=2  IndexOptions=Index vector (dialog)  Indices=[1]  OutputSizes=1
  Selector10 : Selector  InputPortWidth=3  IndexOptions=Index vector (dialog)  Indices=[1 2]  OutputSizes=1
  Selector11 : Selector  InputPortWidth=3  IndexOptions=Index vector (dialog)  Indices=[3]  OutputSizes=1
  Selector2 : Selector  InputPortWidth=2  IndexOptions=Index vector (dialog)  Indices=[1]  OutputSizes=1
  Selector3 : Selector  InputPortWidth=2  IndexOptions=Index vector (dialog)  Indices=[1]  OutputSizes=1
  Selector4 : Selector  InputPortWidth=3  IndexOptions=Index vector (dialog)  Indices=[1 2]  OutputSizes=1
  Selector5 : Selector  InputPortWidth=3  IndexOptions=Index vector (dialog)  Indices=[3]  OutputSizes=1
  Selector6 : Selector  InputPortWidth=3  IndexOptions=Index vector (dialog)  Indices=[3]  OutputSizes=1
  Selector7 : Selector  InputPortWidth=3  IndexOptions=Index vector (dialog)  Indices=[2]  OutputSizes=1
  Selector8 : Selector  InputPortWidth=3  IndexOptions=Index vector (dialog)  Indices=[2]  OutputSizes=1
  Sin : Trigonometry
  Sqrt : Sqrt
  Square : Math  Operator=square
  Square1 : Math  Operator=square
  Sum1 : Sum  Inputs=|-+
  Sum2 : Sum  Inputs=|-+
  Sum{3..6} (4 alike) : Sum  Inputs=|++
  Sum7 : Sum  Inputs=|+-
  Unit Delay : UnitDelay  SampleTime=delay_tilt  HasFrameUpgradeWarning=on
  yaw : Selector  InputPortWidth=3  IndexOptions=Index vector (dialog)  Indices=[3]  OutputSizes=1
  tau_thrust : Outport
  tilt : Outport  Port=2
  tau_pitch : Outport  Port=3
  wires:
  Gain/1 -> MatrixMultiply/2
  Demux2/3 -> Scope/1, tau_pitch/1
  Selector7/1 -> Sum2/2, Cos/1, Gain1/1  "pitch"
  Pitch_ref/1 -> Sum2/1  "pitch_ref"
  Sqrt/1 -> Gain2/1
  Mux/1 -> Gain/1
  Atan2/1 -> Unit Delay/1
  Selector8/1 -> Mux/6  "pitch dot"
  Product/1 -> Sum4/2
  Sum2/1 -> Mux/5
  Reference_Pos/1 -> Selector/1, Selector11/1
  Sum5/1 -> Sqrt/1
  Cos/1 -> Product/1
  Square/1 -> Sum5/2
  Sin/1 -> Product1/2
  Gain1/1 -> Sin/1
  Rate_Current/1 -> Selector8/1
  Product1/1 -> Sum3/2
  Current_Pos/1 -> Selector5/1, Selector4/1
  Demux2/2 -> Sum4/1
  Constant1/1 -> Product/2, Product1/1
  Product2/1 -> Atan2/1
  MatrixMultiply/1 -> Demux2/1
  Selector6/1 -> Mux/4  "vz"
  Sum1/1 -> Mux/1
  Sum7/1 -> Mux/3
  Square1/1 -> Sum5/1
  Current_Attitude/1 -> yaw/1, Selector7/1
  Gain2/1 -> tau_thrust/1
  Demux2/1 -> Sum3/1
  Reciprocal/1 -> Product2/2
  Sum6/1 -> Reciprocal/1
  Constant2/1 -> Sum6/2
  Current_Vel/1 -> Selector10/1, Selector6/1
  Selector5/1 -> Sum7/1  "z"
  Selector11/1 -> Sum7/2  "z_ref"
  Sum4/1 -> Sum6/1, Square/1
  Sum3/1 -> Product2/1, Square1/1
  "Rotation mat "/1(R) -> MatrixMultiply3/1
  Selector/1 -> Selector1/1
  Selector1/1 -> Sum1/1  "x_ref"
  yaw/1 -> "Rotation mat "/1(psi)
  Selector4/1 -> Selector2/1
  Selector2/1 -> Sum1/2  "x"
  MatrixMultiply3/1 -> Selector3/1
  Selector3/1 -> Mux/2  "vx"
  Selector10/1 -> MatrixMultiply3/2
  Constant/1 -> MatrixMultiply/1
  Unit Delay/1 -> tilt/1
